simulink model "tongbukongzhi2"  (R2014b)
settings: Solver=ode45  StartTime=0.0  StopTime=10.0  RelTol=1e-3
undefined symbols (not defined in the file): sigbuilder_block
libraries: simulink x89, fuzblock x41
(part 4 of 5)

== system tongbukongzhi2/Subsystem4/Subsystem3 ==
  In4 : Inport
  In1 : Inport  Port=2
  In2 : Inport  Port=3
  In3 : Inport  Port=4
  Add : Sum  Inputs=+++
  PID Controller1 : simulink/Continuous/PID Controller  Controller=PID  TimeDomain=Continuous-time  SampleTime=-1  IntegratorMethod=Forward Euler  FilterMethod=Forward Euler  Form=Parallel  P=12.9851074749726  I=3.96505413373294  D=0.756963167778154  N=4061.73491108422  InitialConditionSource=internal  InitialConditionForIntegrator=0  InitialConditionForFilter=0  ExternalReset=none  LimitOutput=off  UpperSaturationLimit=inf  LowerSaturationLimit=-inf  LinearizeAsGain=on  AntiWindupMode=none  Kb=1  TrackingMode=off  Kt=1  PParamMin=[]  PParamMax=[]  IParamMin=[]  IParamMax=[]  DParamMin=[]  DParamMax=[]  NParamMin=[]  NParamMax=[]  KbParamMin=[]  KbParamMax=[]  KtParamMin=[]  KtParamMax=[]  POutMin=[]  POutMax=[]  IOutMin=[]  IOutMax=[]  DOutMin=[]  DOutMax=[]  NOutMin=[]  NOutMax=[]  KbOutMin=[]  KbOutMax=[]  KtOutMin=[]  KtOutMax=[]  IntegratorOutMin=[]  IntegratorOutMax=[]  FilterOutMin=[]  FilterOutMax=[]  SumOutMin=[]  SumOutMax=[]  SumI1OutMin=[]  SumI1OutMax=[]  SumI2OutMin=[]  SumI2OutMax=[]  SumI3OutMin=[]  SumI3OutMax=[]  SumDOutMin=[]  SumDOutMax=[]  SaturationOutMin=[]  SaturationOutMax=[]  IntegratorContinuousStateAttributes=''  IntegratorStateMustResolveToSignalObject=off  IntegratorRTWStateStorageClass=Auto  FilterContinuousStateAttributes=''  FilterStateMustResolveToSignalObject=off  FilterRTWStateStorageClass=Auto  DifferentiatorICPrevScaledInput=0  DifferentiatorOutMin=[]  DifferentiatorOutMax=[]  UseFilter=on
  PID Controller2 : simulink/Continuous/PID Controller  Controller=PID  TimeDomain=Continuous-time  SampleTime=-1  IntegratorMethod=Forward Euler  FilterMethod=Forward Euler  Form=Parallel  P=12.9851074749726  I=3.96505413373294  D=0.756963167778154  N=4061.73491108422  InitialConditionSource=internal  InitialConditionForIntegrator=0  InitialConditionForFilter=0  ExternalReset=none  LimitOutput=off  UpperSaturationLimit=inf  LowerSaturationLimit=-inf  LinearizeAsGain=on  AntiWindupMode=none  Kb=1  TrackingMode=off  Kt=1  PParamMin=[]  PParamMax=[]  IParamMin=[]  IParamMax=[]  DParamMin=[]  DParamMax=[]  NParamMin=[]  NParamMax=[]  KbParamMin=[]  KbParamMax=[]  KtParamMin=[]  KtParamMax=[]  POutMin=[]  POutMax=[]  IOutMin=[]  IOutMax=[]  DOutMin=[]  DOutMax=[]  NOutMin=[]  NOutMax=[]  KbOutMin=[]  KbOutMax=[]  KtOutMin=[]  KtOutMax=[]  IntegratorOutMin=[]  IntegratorOutMax=[]  FilterOutMin=[]  FilterOutMax=[]  SumOutMin=[]  SumOutMax=[]  SumI1OutMin=[]  SumI1OutMax=[]  SumI2OutMin=[]  SumI2OutMax=[]  SumI3OutMin=[]  SumI3OutMax=[]  SumDOutMin=[]  SumDOutMax=[]  SaturationOutMin=[]  SaturationOutMax=[]  IntegratorContinuousStateAttributes=''  IntegratorStateMustResolveToSignalObject=off  IntegratorRTWStateStorageClass=Auto  FilterContinuousStateAttributes=''  FilterStateMustResolveToSignalObject=off  FilterRTWStateStorageClass=Auto  DifferentiatorICPrevScaledInput=0  DifferentiatorOutMin=[]  DifferentiatorOutMax=[]  UseFilter=on
  PID Controller5 : simulink/Continuous/PID Controller  Controller=PID  TimeDomain=Continuous-time  SampleTime=-1  IntegratorMethod=Forward Euler  FilterMethod=Forward Euler  Form=Parallel  P=12.9851074749726  I=3.96505413373294  D=0.756963167778154  N=4061.73491108422  InitialConditionSource=internal  InitialConditionForIntegrator=0  InitialConditionForFilter=0  ExternalReset=none  LimitOutput=off  UpperSaturationLimit=inf  LowerSaturationLimit=-inf  LinearizeAsGain=on  AntiWindupMode=none  Kb=1  TrackingMode=off  Kt=1  PParamMin=[]  PParamMax=[]  IParamMin=[]  IParamMax=[]  DParamMin=[]  DParamMax=[]  NParamMin=[]  NParamMax=[]  KbParamMin=[]  KbParamMax=[]  KtParamMin=[]  KtParamMax=[]  POutMin=[]  POutMax=[]  IOutMin=[]  IOutMax=[]  DOutMin=[]  DOutMax=[]  NOutMin=[]  NOutMax=[]  KbOutMin=[]  KbOutMax=[]  KtOutMin=[]  KtOutMax=[]  IntegratorOutMin=[]  IntegratorOutMax=[]  FilterOutMin=[]  FilterOutMax=[]  SumOutMin=[]  SumOutMax=[]  SumI1OutMin=[]  SumI1OutMax=[]  SumI2OutMin=[]  SumI2OutMax=[]  SumI3OutMin=[]  SumI3OutMax=[]  SumDOutMin=[]  SumDOutMax=[]  SaturationOutMin=[]  SaturationOutMax=[]  IntegratorContinuousStateAttributes=''  IntegratorStateMustResolveToSignalObject=off  IntegratorRTWStateStorageClass=Auto  FilterContinuousStateAttributes=''  FilterStateMustResolveToSignalObject=off  FilterRTWStateStorageClass=Auto  DifferentiatorICPrevScaledInput=0  DifferentiatorOutMin=[]  DifferentiatorOutMax=[]  UseFilter=on
  Sum : Sum  Inputs=|+-
  Sum1 : Sum  Inputs=|+-
  Sum2 : Sum  Inputs=|+-
  Out1 : Outport
  wires:
  In4/1 -> Sum/1, Sum1/1, Sum2/1
  In1/1 -> Sum/2
  In2/1 -> Sum1/2
  In3/1 -> Sum2/2
  Sum/1 -> PID Controller1/1
  Sum1/1 -> PID Controller2/1
  Sum2/1 -> PID Controller5/1
  Add/1 -> Out1/1
  PID Controller1/1 -> Add/1
  PID Controller5/1 -> Add/3
  PID Controller2/1 -> Add/2

== system tongbukongzhi2/Subsystem4/Subsystem4 ==
  In1 : Inport
  In2 : Inport  Port=2
  In3 : Inport  Port=3
  In4 : Inport  Port=4
  Add : Sum  Inputs=+++
  PID Controller3 : simulink/Continuous/PID Controller  Controller=PID  TimeDomain=Continuous-time  SampleTime=-1  IntegratorMethod=Forward Euler  FilterMethod=Forward Euler  Form=Parallel  P=27.9924596461686  I=402.197520204602  D=0.419640505495117  N=400.016333492829  InitialConditionSource=internal  InitialConditionForIntegrator=0  InitialConditionForFilter=0  ExternalReset=none  LimitOutput=off  UpperSaturationLimit=inf  LowerSaturationLimit=-inf  LinearizeAsGain=on  AntiWindupMode=none  Kb=1  TrackingMode=off  Kt=1  PParamMin=[]  PParamMax=[]  IParamMin=[]  IParamMax=[]  DParamMin=[]  DParamMax=[]  NParamMin=[]  NParamMax=[]  KbParamMin=[]  KbParamMax=[]  KtParamMin=[]  KtParamMax=[]  POutMin=[]  POutMax=[]  IOutMin=[]  IOutMax=[]  DOutMin=[]  DOutMax=[]  NOutMin=[]  NOutMax=[]  KbOutMin=[]  KbOutMax=[]  KtOutMin=[]  KtOutMax=[]  IntegratorOutMin=[]  IntegratorOutMax=[]  FilterOutMin=[]  FilterOutMax=[]  SumOutMin=[]  SumOutMax=[]  SumI1OutMin=[]  SumI1OutMax=[]  SumI2OutMin=[]  SumI2OutMax=[]  SumI3OutMin=[]  SumI3OutMax=[]  SumDOutMin=[]  SumDOutMax=[]  SaturationOutMin=[]  SaturationOutMax=[]  IntegratorContinuousStateAttributes=''  IntegratorStateMustResolveToSignalObject=off  IntegratorRTWStateStorageClass=Auto  FilterContinuousStateAttributes=''  FilterStateMustResolveToSignalObject=off  FilterRTWStateStorageClass=Auto  DifferentiatorICPrevScaledInput=0  DifferentiatorOutMin=[]  DifferentiatorOutMax=[]  UseFilter=on
  PID Controller4 : simulink/Continuous/PID Controller  Controller=PID  TimeDomain=Continuous-time  SampleTime=-1  IntegratorMethod=Forward Euler  FilterMethod=Forward Euler  Form=Parallel  P=27.9924596461686  I=402.197520204602  D=0.419640505495117  N=400.016333492829  InitialConditionSource=internal  InitialConditionForIntegrator=0  InitialConditionForFilter=0  ExternalReset=none  LimitOutput=off  UpperSaturationLimit=inf  LowerSaturationLimit=-inf  LinearizeAsGain=on  AntiWindupMode=none  Kb=1  TrackingMode=off  Kt=1  PParamMin=[]  PParamMax=[]  IParamMin=[]  IParamMax=[]  DParamMin=[]  DParamMax=[]  NParamMin=[]  NParamMax=[]  KbParamMin=[]  KbParamMax=[]  KtParamMin=[]  KtParamMax=[]  POutMin=[]  POutMax=[]  IOutMin=[]  IOutMax=[]  DOutMin=[]  DOutMax=[]  NOutMin=[]  NOutMax=[]  KbOutMin=[]  KbOutMax=[]  KtOutMin=[]  KtOutMax=[]  IntegratorOutMin=[]  IntegratorOutMax=[]  FilterOutMin=[]  FilterOutMax=[]  SumOutMin=[]  SumOutMax=[]  SumI1OutMin=[]  SumI1OutMax=[]  SumI2OutMin=[]  SumI2OutMax=[]  SumI3OutMin=[]  SumI3OutMax=[]  SumDOutMin=[]  SumDOutMax=[]  SaturationOutMin=[]  SaturationOutMax=[]  IntegratorContinuousStateAttributes=''  IntegratorStateMustResolveToSignalObject=off  IntegratorRTWStateStorageClass=Auto  FilterContinuousStateAttributes=''  FilterStateMustResolveToSignalObject=off  FilterRTWStateStorageClass=Auto  DifferentiatorICPrevScaledInput=0  DifferentiatorOutMin=[]  DifferentiatorOutMax=[]  UseFilter=on
  PID Controller6 : simulink/Continuous/PID Controller  Controller=PID  TimeDomain=Continuous-time  SampleTime=-1  IntegratorMethod=Forward Euler  FilterMethod=Forward Euler  Form=Parallel  P=27.9924596461686  I=402.197520204602  D=0.419640505495117  N=400.016333492829  InitialConditionSource=internal  InitialConditionForIntegrator=0  InitialConditionForFilter=0  ExternalReset=none  LimitOutput=off  UpperSaturationLimit=inf  LowerSaturationLimit=-inf  LinearizeAsGain=on  AntiWindupMode=none  Kb=1  TrackingMode=off  Kt=1  PParamMin=[]  PParamMax=[]  IParamMin=[]  IParamMax=[]  DParamMin=[]  DParamMax=[]  NParamMin=[]  NParamMax=[]  KbParamMin=[]  KbParamMax=[]  KtParamMin=[]  KtParamMax=[]  POutMin=[]  POutMax=[]  IOutMin=[]  IOutMax=[]  DOutMin=[]  DOutMax=[]  NOutMin=[]  NOutMax=[]  KbOutMin=[]  KbOutMax=[]  KtOutMin=[]  KtOutMax=[]  IntegratorOutMin=[]  IntegratorOutMax=[]  FilterOutMin=[]  FilterOutMax=[]  SumOutMin=[]  SumOutMax=[]  SumI1OutMin=[]  SumI1OutMax=[]  SumI2OutMin=[]  SumI2OutMax=[]  SumI3OutMin=[]  SumI3OutMax=[]  SumDOutMin=[]  SumDOutMax=[]  SaturationOutMin=[]  SaturationOutMax=[]  IntegratorContinuousStateAttributes=''  IntegratorStateMustResolveToSignalObject=off  IntegratorRTWStateStorageClass=Auto  FilterContinuousStateAttributes=''  FilterStateMustResolveToSignalObject=off  FilterRTWStateStorageClass=Auto  DifferentiatorICPrevScaledInput=0  DifferentiatorOutMin=[]  DifferentiatorOutMax=[]  UseFilter=on
  Sum : Sum  Inputs=|+-
  Sum1 : Sum  Inputs=|+-
  Sum2 : Sum  Inputs=|+-
  Out1 : Outport
  wires:
  In1/1 -> Sum/1, Sum1/1, Sum2/1
  In2/1 -> Sum/2
  In3/1 -> Sum1/2
  In4/1 -> Sum2/2
  Sum/1 -> PID Controller3/1
  Sum1/1 -> PID Controller4/1
  Sum2/1 -> PID Controller6/1
  Add/1 -> Out1/1
  PID Controller3/1 -> Add/1
  PID Controller4/1 -> Add/2
  PID Controller6/1 -> Add/3

== system tongbukongzhi2/Subsystem4/Subsystem5 ==
  In2 : Inport
  In1 : Inport  Port=2
  In3 : Inport  Port=3
  In4 : Inport  Port=4
  Add : Sum  Inputs=+++
  PID Controller1 : simulink/Continuous/PID Controller  Controller=PID  TimeDomain=Continuous-time  SampleTime=-1  IntegratorMethod=Forward Euler  FilterMethod=Forward Euler  Form=Parallel  P=27.9924596461686  I=402.197520204602  D=0.419640505495117  N=400.016333492829  InitialConditionSource=internal  InitialConditionForIntegrator=0  InitialConditionForFilter=0  ExternalReset=none  LimitOutput=off  UpperSaturationLimit=inf  LowerSaturationLimit=-inf  LinearizeAsGain=on  AntiWindupMode=none  Kb=1  TrackingMode=off  Kt=1  PParamMin=[]  PParamMax=[]  IParamMin=[]  IParamMax=[]  DParamMin=[]  DParamMax=[]  NParamMin=[]  NParamMax=[]  KbParamMin=[]  KbParamMax=[]  KtParamMin=[]  KtParamMax=[]  POutMin=[]  POutMax=[]  IOutMin=[]  IOutMax=[]  DOutMin=[]  DOutMax=[]  NOutMin=[]  NOutMax=[]  KbOutMin=[]  KbOutMax=[]  KtOutMin=[]  KtOutMax=[]  IntegratorOutMin=[]  IntegratorOutMax=[]  FilterOutMin=[]  FilterOutMax=[]  SumOutMin=[]  SumOutMax=[]  SumI1OutMin=[]  SumI1OutMax=[]  SumI2OutMin=[]  SumI2OutMax=[]  SumI3OutMin=[]  SumI3OutMax=[]  SumDOutMin=[]  SumDOutMax=[]  SaturationOutMin=[]  SaturationOutMax=[]  IntegratorContinuousStateAttributes=''  IntegratorStateMustResolveToSignalObject=off  IntegratorRTWStateStorageClass=Auto  FilterContinuousStateAttributes=''  FilterStateMustResolveToSignalObject=off  FilterRTWStateStorageClass=Auto  DifferentiatorICPrevScaledInput=0  DifferentiatorOutMin=[]  DifferentiatorOutMax=[]  UseFilter=on
  PID Controller2 : simulink/Continuous/PID Controller  Controller=PID  TimeDomain=Continuous-time  SampleTime=-1  IntegratorMethod=Forward Euler  FilterMethod=Forward Euler  Form=Parallel  P=27.9924596461686  I=402.197520204602  D=0.419640505495117  N=400.016333492829  InitialConditionSource=internal  InitialConditionForIntegrator=0  InitialConditionForFilter=0  ExternalReset=none  LimitOutput=off  UpperSaturationLimit=inf  LowerSaturationLimit=-inf  LinearizeAsGain=on  AntiWindupMode=none  Kb=1  TrackingMode=off  Kt=1  PParamMin=[]  PParamMax=[]  IParamMin=[]  IParamMax=[]  DParamMin=[]  DParamMax=[]  NParamMin=[]  NParamMax=[]  KbParamMin=[]  KbParamMax=[]  KtParamMin=[]  KtParamMax=[]  POutMin=[]  POutMax=[]  IOutMin=[]  IOutMax=[]  DOutMin=[]  DOutMax=[]  NOutMin=[]  NOutMax=[]  KbOutMin=[]  KbOutMax=[]  KtOutMin=[]  KtOutMax=[]  IntegratorOutMin=[]  IntegratorOutMax=[]  FilterOutMin=[]  FilterOutMax=[]  SumOutMin=[]  SumOutMax=[]  SumI1OutMin=[]  SumI1OutMax=[]  SumI2OutMin=[]  SumI2OutMax=[]  SumI3OutMin=[]  SumI3OutMax=[]  SumDOutMin=[]  SumDOutMax=[]  SaturationOutMin=[]  SaturationOutMax=[]  IntegratorContinuousStateAttributes=''  IntegratorStateMustResolveToSignalObject=off  IntegratorRTWStateStorageClass=Auto  FilterContinuousStateAttributes=''  FilterStateMustResolveToSignalObject=off  FilterRTWStateStorageClass=Auto  DifferentiatorICPrevScaledInput=0  DifferentiatorOutMin=[]  DifferentiatorOutMax=[]  UseFilter=on
  PID Controller5 : simulink/Continuous/PID Controller  Controller=PID  TimeDomain=Continuous-time  SampleTime=-1  IntegratorMethod=Forward Euler  FilterMethod=Forward Euler  Form=Parallel  P=27.9924596461686  I=402.197520204602  D=0.419640505495117  N=400.016333492829  InitialConditionSource=internal  InitialConditionForIntegrator=0  InitialConditionForFilter=0  ExternalReset=none  LimitOutput=off  UpperSaturationLimit=inf  LowerSaturationLimit=-inf  LinearizeAsGain=on  AntiWindupMode=none  Kb=1  TrackingMode=off  Kt=1  PParamMin=[]  PParamMax=[]  IParamMin=[]  IParamMax=[]  DParamMin=[]  DParamMax=[]  NParamMin=[]  NParamMax=[]  KbParamMin=[]  KbParamMax=[]  KtParamMin=[]  KtParamMax=[]  POutMin=[]  POutMax=[]  IOutMin=[]  IOutMax=[]  DOutMin=[]  DOutMax=[]  NOutMin=[]  NOutMax=[]  KbOutMin=[]  KbOutMax=[]  KtOutMin=[]  KtOutMax=[]  IntegratorOutMin=[]  IntegratorOutMax=[]  FilterOutMin=[]  FilterOutMax=[]  SumOutMin=[]  SumOutMax=[]  SumI1OutMin=[]  SumI1OutMax=[]  SumI2OutMin=[]  SumI2OutMax=[]  SumI3OutMin=[]  SumI3OutMax=[]  SumDOutMin=[]  SumDOutMax=[]  SaturationOutMin=[]  SaturationOutMax=[]  IntegratorContinuousStateAttributes=''  IntegratorStateMustResolveToSignalObject=off  IntegratorRTWStateStorageClass=Auto  FilterContinuousStateAttributes=''  FilterStateMustResolveToSignalObject=off  FilterRTWStateStorageClass=Auto  DifferentiatorICPrevScaledInput=0  DifferentiatorOutMin=[]  DifferentiatorOutMax=[]  UseFilter=on
  Sum : Sum  Inputs=|+-
  Sum1 : Sum  Inputs=|+-
  Sum2 : Sum  Inputs=|+-
  Out1 : Outport
  wires:
  In2/1 -> Sum/1, Sum1/1, Sum2/1
  In1/1 -> Sum/2
  In3/1 -> Sum1/2
  In4/1 -> Sum2/2
  Sum/1 -> PID Controller1/1
  Sum1/1 -> PID Controller2/1
  Sum2/1 -> PID Controller5/1
  Add/1 -> Out1/1
  PID Controller1/1 -> Add/1
  PID Controller2/1 -> Add/2
  PID Controller5/1 -> Add/3

== system tongbukongzhi2/Subsystem4/Subsystem6 ==
  In3 : Inport
  In1 : Inport  Port=2
  In2 : Inport  Port=3
  In4 : Inport  Port=4
  Add : Sum  Inputs=+++
  PID Controller1 : simulink/Continuous/PID Controller  Controller=PID  TimeDomain=Continuous-time  SampleTime=-1  IntegratorMethod=Forward Euler  FilterMethod=Forward Euler  Form=Parallel  P=27.9924596461686  I=402.197520204602  D=0.419640505495117  N=400.016333492829  InitialConditionSource=internal  InitialConditionForIntegrator=0  InitialConditionForFilter=0  ExternalReset=none  LimitOutput=off  UpperSaturationLimit=inf  LowerSaturationLimit=-inf  LinearizeAsGain=on  AntiWindupMode=none  Kb=1  TrackingMode=off  Kt=1  PParamMin=[]  PParamMax=[]  IParamMin=[]  IParamMax=[]  DParamMin=[]  DParamMax=[]  NParamMin=[]  NParamMax=[]  KbParamMin=[]  KbParamMax=[]  KtParamMin=[]  KtParamMax=[]  POutMin=[]  POutMax=[]  IOutMin=[]  IOutMax=[]  DOutMin=[]  DOutMax=[]  NOutMin=[]  NOutMax=[]  KbOutMin=[]  KbOutMax=[]  KtOutMin=[]  KtOutMax=[]  IntegratorOutMin=[]  IntegratorOutMax=[]  FilterOutMin=[]  FilterOutMax=[]  SumOutMin=[]  SumOutMax=[]  SumI1OutMin=[]  SumI1OutMax=[]  SumI2OutMin=[]  SumI2OutMax=[]  SumI3OutMin=[]  SumI3OutMax=[]  SumDOutMin=[]  SumDOutMax=[]  SaturationOutMin=[]  SaturationOutMax=[]  IntegratorContinuousStateAttributes=''  IntegratorStateMustResolveToSignalObject=off  IntegratorRTWStateStorageClass=Auto  FilterContinuousStateAttributes=''  FilterStateMustResolveToSignalObject=off  FilterRTWStateStorageClass=Auto  DifferentiatorICPrevScaledInput=0  DifferentiatorOutMin=[]  DifferentiatorOutMax=[]  UseFilter=on
  PID Controller2 : simulink/Continuous/PID Controller  Controller=PID  TimeDomain=Continuous-time  SampleTime=-1  IntegratorMethod=Forward Euler  FilterMethod=Forward Euler  Form=Parallel  P=27.9924596461686  I=402.197520204602  D=0.419640505495117  N=400.016333492829  InitialConditionSource=internal  InitialConditionForIntegrator=0  InitialConditionForFilter=0  ExternalReset=none  LimitOutput=off  UpperSaturationLimit=inf  LowerSaturationLimit=-inf  LinearizeAsGain=on  AntiWindupMode=none  Kb=1  TrackingMode=off  Kt=1  PParamMin=[]  PParamMax=[]  IParamMin=[]  IParamMax=[]  DParamMin=[]  DParamMax=[]  NParamMin=[]  NParamMax=[]  KbParamMin=[]  KbParamMax=[]  KtParamMin=[]  KtParamMax=[]  POutMin=[]  POutMax=[]  IOutMin=[]  IOutMax=[]  DOutMin=[]  DOutMax=[]  NOutMin=[]  NOutMax=[]  KbOutMin=[]  KbOutMax=[]  KtOutMin=[]  KtOutMax=[]  IntegratorOutMin=[]  IntegratorOutMax=[]  FilterOutMin=[]  FilterOutMax=[]  SumOutMin=[]  SumOutMax=[]  SumI1OutMin=[]  SumI1OutMax=[]  SumI2OutMin=[]  SumI2OutMax=[]  SumI3OutMin=[]  SumI3OutMax=[]  SumDOutMin=[]  SumDOutMax=[]  SaturationOutMin=[]  SaturationOutMax=[]  IntegratorContinuousStateAttributes=''  IntegratorStateMustResolveToSignalObject=off  IntegratorRTWStateStorageClass=Auto  FilterContinuousStateAttributes=''  FilterStateMustResolveToSignalObject=off  FilterRTWStateStorageClass=Auto  DifferentiatorICPrevScaledInput=0  DifferentiatorOutMin=[]  DifferentiatorOutMax=[]  UseFilter=on
  PID Controller3 : simulink/Continuous/PID Controller  Controller=PID  TimeDomain=Continuous-time  SampleTime=-1  IntegratorMethod=Forward Euler  FilterMethod=Forward Euler  Form=Parallel  P=27.9924596461686  I=402.197520204602  D=0.419640505495117  N=400.016333492829  InitialConditionSource=internal  InitialConditionForIntegrator=0  InitialConditionForFilter=0  ExternalReset=none  LimitOutput=off  UpperSaturationLimit=inf  LowerSaturationLimit=-inf  LinearizeAsGain=on  AntiWindupMode=none  Kb=1  TrackingMode=off  Kt=1  PParamMin=[]  PParamMax=[]  IParamMin=[]  IParamMax=[]  DParamMin=[]  DParamMax=[]  NParamMin=[]  NParamMax=[]  KbParamMin=[]  KbParamMax=[]  KtParamMin=[]  KtParamMax=[]  POutMin=[]  POutMax=[]  IOutMin=[]  IOutMax=[]  DOutMin=[]  DOutMax=[]  NOutMin=[]  NOutMax=[]  KbOutMin=[]  KbOutMax=[]  KtOutMin=[]  KtOutMax=[]  IntegratorOutMin=[]  IntegratorOutMax=[]  FilterOutMin=[]  FilterOutMax=[]  SumOutMin=[]  SumOutMax=[]  SumI1OutMin=[]  SumI1OutMax=[]  SumI2OutMin=[]  SumI2OutMax=[]  SumI3OutMin=[]  SumI3OutMax=[]  SumDOutMin=[]  SumDOutMax=[]  SaturationOutMin=[]  SaturationOutMax=[]  IntegratorContinuousStateAttributes=''  IntegratorStateMustResolveToSignalObject=off  IntegratorRTWStateStorageClass=Auto  FilterContinuousStateAttributes=''  FilterStateMustResolveToSignalObject=off  FilterRTWStateStorageClass=Auto  DifferentiatorICPrevScaledInput=0  DifferentiatorOutMin=[]  DifferentiatorOutMax=[]  UseFilter=on
  Sum : Sum  Inputs=|+-
  Sum1 : Sum  Inputs=|+-
  Sum2 : Sum  Inputs=|+-
  Out1 : Outport
  wires:
  In3/1 -> Sum/1, Sum1/1, Sum2/1
  In1/1 -> Sum/2
  In2/1 -> Sum1/2
  In4/1 -> Sum2/2
  Sum/1 -> PID Controller1/1
  Sum1/1 -> PID Controller2/1
  Sum2/1 -> PID Controller3/1
  Add/1 -> Out1/1
  PID Controller1/1 -> Add/1
  PID Controller2/1 -> Add/2
  PID Controller3/1 -> Add/3

== system tongbukongzhi2/Subsystem4/Subsystem7 ==
  In4 : Inport
  In1 : Inport  Port=2
  In2 : Inport  Port=3
  In3 : Inport  Port=4
  Add : Sum  Inputs=+++
  PID Controller3 : simulink/Continuous/PID Controller  Controller=PID  TimeDomain=Continuous-time  SampleTime=-1  IntegratorMethod=Forward Euler  FilterMethod=Forward Euler  Form=Parallel  P=27.9924596461686  I=402.197520204602  D=0.419640505495117  N=400.016333492829  InitialConditionSource=internal  InitialConditionForIntegrator=0  InitialConditionForFilter=0  ExternalReset=none  LimitOutput=off  UpperSaturationLimit=inf  LowerSaturationLimit=-inf  LinearizeAsGain=on  AntiWindupMode=none  Kb=1  TrackingMode=off  Kt=1  PParamMin=[]  PParamMax=[]  IParamMin=[]  IParamMax=[]  DParamMin=[]  DParamMax=[]  NParamMin=[]  NParamMax=[]  KbParamMin=[]  KbParamMax=[]  KtParamMin=[]  KtParamMax=[]  POutMin=[]  POutMax=[]  IOutMin=[]  IOutMax=[]  DOutMin=[]  DOutMax=[]  NOutMin=[]  NOutMax=[]  KbOutMin=[]  KbOutMax=[]  KtOutMin=[]  KtOutMax=[]  IntegratorOutMin=[]  IntegratorOutMax=[]  FilterOutMin=[]  FilterOutMax=[]  SumOutMin=[]  SumOutMax=[]  SumI1OutMin=[]  SumI1OutMax=[]  SumI2OutMin=[]  SumI2OutMax=[]  SumI3OutMin=[]  SumI3OutMax=[]  SumDOutMin=[]  SumDOutMax=[]  SaturationOutMin=[]  SaturationOutMax=[]  IntegratorContinuousStateAttributes=''  IntegratorStateMustResolveToSignalObject=off  IntegratorRTWStateStorageClass=Auto  FilterContinuousStateAttributes=''  FilterStateMustResolveToSignalObject=off  FilterRTWStateStorageClass=Auto  DifferentiatorICPrevScaledInput=0  DifferentiatorOutMin=[]  DifferentiatorOutMax=[]  UseFilter=on
  PID Controller4 : simulink/Continuous/PID Controller  Controller=PID  TimeDomain=Continuous-time  SampleTime=-1  IntegratorMethod=Forward Euler  FilterMethod=Forward Euler  Form=Parallel  P=27.9924596461686  I=402.197520204602  D=0.419640505495117  N=400.016333492829  InitialConditionSource=internal  InitialConditionForIntegrator=0  InitialConditionForFilter=0  ExternalReset=none  LimitOutput=off  UpperSaturationLimit=inf  LowerSaturationLimit=-inf  LinearizeAsGain=on  AntiWindupMode=none  Kb=1  TrackingMode=off  Kt=1  PParamMin=[]  PParamMax=[]  IParamMin=[]  IParamMax=[]  DParamMin=[]  DParamMax=[]  NParamMin=[]  NParamMax=[]  KbParamMin=[]  KbParamMax=[]  KtParamMin=[]  KtParamMax=[]  POutMin=[]  POutMax=[]  IOutMin=[]  IOutMax=[]  DOutMin=[]  DOutMax=[]  NOutMin=[]  NOutMax=[]  KbOutMin=[]  KbOutMax=[]  KtOutMin=[]  KtOutMax=[]  IntegratorOutMin=[]  IntegratorOutMax=[]  FilterOutMin=[]  FilterOutMax=[]  SumOutMin=[]  SumOutMax=[]  SumI1OutMin=[]  SumI1OutMax=[]  SumI2OutMin=[]  SumI2OutMax=[]  SumI3OutMin=[]  SumI3OutMax=[]  SumDOutMin=[]  SumDOutMax=[]  SaturationOutMin=[]  SaturationOutMax=[]  IntegratorContinuousStateAttributes=''  IntegratorStateMustResolveToSignalObject=off  IntegratorRTWStateStorageClass=Auto  FilterContinuousStateAttributes=''  FilterStateMustResolveToSignalObject=off  FilterRTWStateStorageClass=Auto  DifferentiatorICPrevScaledInput=0  DifferentiatorOutMin=[]  DifferentiatorOutMax=[]  UseFilter=on
  PID Controller6 : simulink/Continuous/PID Controller  Controller=PID  TimeDomain=Continuous-time  SampleTime=-1  IntegratorMethod=Forward Euler  FilterMethod=Forward Euler  Form=Parallel  P=27.9924596461686  I=402.197520204602  D=0.419640505495117  N=400.016333492829  InitialConditionSource=internal  InitialConditionForIntegrator=0  InitialConditionForFilter=0  ExternalReset=none  LimitOutput=off  UpperSaturationLimit=inf  LowerSaturationLimit=-inf  LinearizeAsGain=on  AntiWindupMode=none  Kb=1  TrackingMode=off  Kt=1  PParamMin=[]  PParamMax=[]  IParamMin=[]  IParamMax=[]  DParamMin=[]  DParamMax=[]  NParamMin=[]  NParamMax=[]  KbParamMin=[]  KbParamMax=[]  KtParamMin=[]  KtParamMax=[]  POutMin=[]  POutMax=[]  IOutMin=[]  IOutMax=[]  DOutMin=[]  DOutMax=[]  NOutMin=[]  NOutMax=[]  KbOutMin=[]  KbOutMax=[]  KtOutMin=[]  KtOutMax=[]  IntegratorOutMin=[]  IntegratorOutMax=[]  FilterOutMin=[]  FilterOutMax=[]  SumOutMin=[]  SumOutMax=[]  SumI1OutMin=[]  SumI1OutMax=[]  SumI2OutMin=[]  SumI2OutMax=[]  SumI3OutMin=[]  SumI3OutMax=[]  SumDOutMin=[]  SumDOutMax=[]  SaturationOutMin=[]  SaturationOutMax=[]  IntegratorContinuousStateAttributes=''  IntegratorStateMustResolveToSignalObject=off  IntegratorRTWStateStorageClass=Auto  FilterContinuousStateAttributes=''  FilterStateMustResolveToSignalObject=off  FilterRTWStateStorageClass=Auto  DifferentiatorICPrevScaledInput=0  DifferentiatorOutMin=[]  DifferentiatorOutMax=[]  UseFilter=on
  Sum : Sum  Inputs=|+-
  Sum1 : Sum  Inputs=|+-
  Sum2 : Sum  Inputs=|+-
  Out1 : Outport
  wires:
  In4/1 -> Sum/1, Sum1/1, Sum2/1
  In1/1 -> Sum/2
  In2/1 -> Sum1/2
  In3/1 -> Sum2/2
  Sum/1 -> PID Controller3/1
  Sum1/1 -> PID Controller4/1
  Sum2/1 -> PID Controller6/1
  Add/1 -> Out1/1
  PID Controller3/1 -> Add/1
  PID Controller6/1 -> Add/3
  PID Controller4/1 -> Add/2

== system tongbukongzhi2/Subsystem4/Subsystem8 ==
  In1 : Inport
  In2 : Inport  Port=2
  In3 : Inport  Port=3
  In4 : Inport  Port=4
  Add : Sum  Inputs=+++
  PID Controller4 : simulink/Continuous/PID Controller  Controller=PID  TimeDomain=Continuous-time  SampleTime=-1  IntegratorMethod=Forward Euler  FilterMethod=Forward Euler  Form=Parallel  P=1.70949141415732  I=21.1355731705013  D=-0.019753461495741  N=20.6090721378652  InitialConditionSource=internal  InitialConditionForIntegrator=0  InitialConditionForFilter=0  ExternalReset=none  LimitOutput=off  UpperSaturationLimit=inf  LowerSaturationLimit=-inf  LinearizeAsGain=on  AntiWindupMode=none  Kb=1  TrackingMode=off  Kt=1  PParamMin=[]  PParamMax=[]  IParamMin=[]  IParamMax=[]  DParamMin=[]  DParamMax=[]  NParamMin=[]  NParamMax=[]  KbParamMin=[]  KbParamMax=[]  KtParamMin=[]  KtParamMax=[]  POutMin=[]  POutMax=[]  IOutMin=[]  IOutMax=[]  DOutMin=[]  DOutMax=[]  NOutMin=[]  NOutMax=[]  KbOutMin=[]  KbOutMax=[]  KtOutMin=[]  KtOutMax=[]  IntegratorOutMin=[]  IntegratorOutMax=[]  FilterOutMin=[]  FilterOutMax=[]  SumOutMin=[]  SumOutMax=[]  SumI1OutMin=[]  SumI1OutMax=[]  SumI2OutMin=[]  SumI2OutMax=[]  SumI3OutMin=[]  SumI3OutMax=[]  SumDOutMin=[]  SumDOutMax=[]  SaturationOutMin=[]  SaturationOutMax=[]  IntegratorContinuousStateAttributes=''  IntegratorStateMustResolveToSignalObject=off  IntegratorRTWStateStorageClass=Auto  FilterContinuousStateAttributes=''  FilterStateMustResolveToSignalObject=off  FilterRTWStateStorageClass=Auto  DifferentiatorICPrevScaledInput=0  DifferentiatorOutMin=[]  DifferentiatorOutMax=[]  UseFilter=on
  PID Controller5 : simulink/Continuous/PID Controller  Controller=PID  TimeDomain=Continuous-time  SampleTime=-1  IntegratorMethod=Forward Euler  FilterMethod=Forward Euler  Form=Parallel  P=1.70949141415732  I=21.1355731705013  D=-0.019753461495741  N=20.6090721378652  InitialConditionSource=internal  InitialConditionForIntegrator=0  InitialConditionForFilter=0  ExternalReset=none  LimitOutput=off  UpperSaturationLimit=inf  LowerSaturationLimit=-inf  LinearizeAsGain=on  AntiWindupMode=none  Kb=1  TrackingMode=off  Kt=1  PParamMin=[]  PParamMax=[]  IParamMin=[]  IParamMax=[]  DParamMin=[]  DParamMax=[]  NParamMin=[]  NParamMax=[]  KbParamMin=[]  KbParamMax=[]  KtParamMin=[]  KtParamMax=[]  POutMin=[]  POutMax=[]  IOutMin=[]  IOutMax=[]  DOutMin=[]  DOutMax=[]  NOutMin=[]  NOutMax=[]  KbOutMin=[]  KbOutMax=[]  KtOutMin=[]  KtOutMax=[]  IntegratorOutMin=[]  IntegratorOutMax=[]  FilterOutMin=[]  FilterOutMax=[]  SumOutMin=[]  SumOutMax=[]  SumI1OutMin=[]  SumI1OutMax=[]  SumI2OutMin=[]  SumI2OutMax=[]  SumI3OutMin=[]  SumI3OutMax=[]  SumDOutMin=[]  SumDOutMax=[]  SaturationOutMin=[]  SaturationOutMax=[]  IntegratorContinuousStateAttributes=''  IntegratorStateMustResolveToSignalObject=off  IntegratorRTWStateStorageClass=Auto  FilterContinuousStateAttributes=''  FilterStateMustResolveToSignalObject=off  FilterRTWStateStorageClass=Auto  DifferentiatorICPrevScaledInput=0  DifferentiatorOutMin=[]  DifferentiatorOutMax=[]  UseFilter=on
  PID Controller6 : simulink/Continuous/PID Controller  Controller=PID  TimeDomain=Continuous-time  SampleTime=-1  IntegratorMethod=Forward Euler  FilterMethod=Forward Euler  Form=Parallel  P=1.70949141415732  I=21.1355731705013  D=-0.019753461495741  N=20.6090721378652  InitialConditionSource=internal  InitialConditionForIntegrator=0  InitialConditionForFilter=0  ExternalReset=none  LimitOutput=off  UpperSaturationLimit=inf  LowerSaturationLimit=-inf  LinearizeAsGain=on  AntiWindupMode=none  Kb=1  TrackingMode=off  Kt=1  PParamMin=[]  PParamMax=[]  IParamMin=[]  IParamMax=[]  DParamMin=[]  DParamMax=[]  NParamMin=[]  NParamMax=[]  KbParamMin=[]  KbParamMax=[]  KtParamMin=[]  KtParamMax=[]  POutMin=[]  POutMax=[]  IOutMin=[]  IOutMax=[]  DOutMin=[]  DOutMax=[]  NOutMin=[]  NOutMax=[]  KbOutMin=[]  KbOutMax=[]  KtOutMin=[]  KtOutMax=[]  IntegratorOutMin=[]  IntegratorOutMax=[]  FilterOutMin=[]  FilterOutMax=[]  SumOutMin=[]  SumOutMax=[]  SumI1OutMin=[]  SumI1OutMax=[]  SumI2OutMin=[]  SumI2OutMax=[]  SumI3OutMin=[]  SumI3OutMax=[]  SumDOutMin=[]  SumDOutMax=[]  SaturationOutMin=[]  SaturationOutMax=[]  IntegratorContinuousStateAttributes=''  IntegratorStateMustResolveToSignalObject=off  IntegratorRTWStateStorageClass=Auto  FilterContinuousStateAttributes=''  FilterStateMustResolveToSignalObject=off  FilterRTWStateStorageClass=Auto  DifferentiatorICPrevScaledInput=0  DifferentiatorOutMin=[]  DifferentiatorOutMax=[]  UseFilter=on
  Sum : Sum  Inputs=|+-
  Sum1 : Sum  Inputs=|+-
  Sum2 : Sum  Inputs=|+-
  Out1 : Outport
  wires:
  In1/1 -> Sum/1, Sum1/1, Sum2/1
  In2/1 -> Sum/2
  In3/1 -> Sum1/2
  In4/1 -> Sum2/2
  Sum/1 -> PID Controller4/1
  Sum1/1 -> PID Controller5/1
  Sum2/1 -> PID Controller6/1
  Add/1 -> Out1/1
  PID Controller4/1 -> Add/1
  PID Controller5/1 -> Add/2
  PID Controller6/1 -> Add/3

== system tongbukongzhi2/Subsystem4/Subsystem9 ==
  In2 : Inport
  In1 : Inport  Port=2
  In3 : Inport  Port=3
  In4 : Inport  Port=4
  Add : Sum  Inputs=+++
  PID Controller4 : simulink/Continuous/PID Controller  Controller=PID  TimeDomain=Continuous-time  SampleTime=-1  IntegratorMethod=Forward Euler  FilterMethod=Forward Euler  Form=Parallel  P=1.70949141415732  I=21.1355731705013  D=-0.019753461495741  N=20.6090721378652  InitialConditionSource=internal  InitialConditionForIntegrator=0  InitialConditionForFilter=0  ExternalReset=none  LimitOutput=off  UpperSaturationLimit=inf  LowerSaturationLimit=-inf  LinearizeAsGain=on  AntiWindupMode=none  Kb=1  TrackingMode=off  Kt=1  PParamMin=[]  PParamMax=[]  IParamMin=[]  IParamMax=[]  DParamMin=[]  DParamMax=[]  NParamMin=[]  NParamMax=[]  KbParamMin=[]  KbParamMax=[]  KtParamMin=[]  KtParamMax=[]  POutMin=[]  POutMax=[]  IOutMin=[]  IOutMax=[]  DOutMin=[]  DOutMax=[]  NOutMin=[]  NOutMax=[]  KbOutMin=[]  KbOutMax=[]  KtOutMin=[]  KtOutMax=[]  IntegratorOutMin=[]  IntegratorOutMax=[]  FilterOutMin=[]  FilterOutMax=[]  SumOutMin=[]  SumOutMax=[]  SumI1OutMin=[]  SumI1OutMax=[]  SumI2OutMin=[]  SumI2OutMax=[]  SumI3OutMin=[]  SumI3OutMax=[]  SumDOutMin=[]  SumDOutMax=[]  SaturationOutMin=[]  SaturationOutMax=[]  IntegratorContinuousStateAttributes=''  IntegratorStateMustResolveToSignalObject=off  IntegratorRTWStateStorageClass=Auto  FilterContinuousStateAttributes=''  FilterStateMustResolveToSignalObject=off  FilterRTWStateStorageClass=Auto  DifferentiatorICPrevScaledInput=0  DifferentiatorOutMin=[]  DifferentiatorOutMax=[]  UseFilter=on
  PID Controller5 : simulink/Continuous/PID Controller  Controller=PID  TimeDomain=Continuous-time  SampleTime=-1  IntegratorMethod=Forward Euler  FilterMethod=Forward Euler  Form=Parallel  P=1.70949141415732  I=21.1355731705013  D=-0.019753461495741  N=20.6090721378652  InitialConditionSource=internal  InitialConditionForIntegrator=0  InitialConditionForFilter=0  ExternalReset=none  LimitOutput=off  UpperSaturationLimit=inf  LowerSaturationLimit=-inf  LinearizeAsGain=on  AntiWindupMode=none  Kb=1  TrackingMode=off  Kt=1  PParamMin=[]  PParamMax=[]  IParamMin=[]  IParamMax=[]  DParamMin=[]  DParamMax=[]  NParamMin=[]  NParamMax=[]  KbParamMin=[]  KbParamMax=[]  KtParamMin=[]  KtParamMax=[]  POutMin=[]  POutMax=[]  IOutMin=[]  IOutMax=[]  DOutMin=[]  DOutMax=[]  NOutMin=[]  NOutMax=[]  KbOutMin=[]  KbOutMax=[]  KtOutMin=[]  KtOutMax=[]  IntegratorOutMin=[]  IntegratorOutMax=[]  FilterOutMin=[]  FilterOutMax=[]  SumOutMin=[]  SumOutMax=[]  SumI1OutMin=[]  SumI1OutMax=[]  SumI2OutMin=[]  SumI2OutMax=[]  SumI3OutMin=[]  SumI3OutMax=[]  SumDOutMin=[]  SumDOutMax=[]  SaturationOutMin=[]  SaturationOutMax=[]  IntegratorContinuousStateAttributes=''  IntegratorStateMustResolveToSignalObject=off  IntegratorRTWStateStorageClass=Auto  FilterContinuousStateAttributes=''  FilterStateMustResolveToSignalObject=off  FilterRTWStateStorageClass=Auto  DifferentiatorICPrevScaledInput=0  DifferentiatorOutMin=[]  DifferentiatorOutMax=[]  UseFilter=on
  PID Controller6 : simulink/Continuous/PID Controller  Controller=PID  TimeDomain=Continuous-time  SampleTime=-1  IntegratorMethod=Forward Euler  FilterMethod=Forward Euler  Form=Parallel  P=1.70949141415732  I=21.1355731705013  D=-0.019753461495741  N=20.6090721378652  InitialConditionSource=internal  InitialConditionForIntegrator=0  InitialConditionForFilter=0  ExternalReset=none  LimitOutput=off  UpperSaturationLimit=inf  LowerSaturationLimit=-inf  LinearizeAsGain=on  AntiWindupMode=none  Kb=1  TrackingMode=off  Kt=1  PParamMin=[]  PParamMax=[]  IParamMin=[]  IParamMax=[]  DParamMin=[]  DParamMax=[]  NParamMin=[]  NParamMax=[]  KbParamMin=[]  KbParamMax=[]  KtParamMin=[]  KtParamMax=[]  POutMin=[]  POutMax=[]  IOutMin=[]  IOutMax=[]  DOutMin=[]  DOutMax=[]  NOutMin=[]  NOutMax=[]  KbOutMin=[]  KbOutMax=[]  KtOutMin=[]  KtOutMax=[]  IntegratorOutMin=[]  IntegratorOutMax=[]  FilterOutMin=[]  FilterOutMax=[]  SumOutMin=[]  SumOutMax=[]  SumI1OutMin=[]  SumI1OutMax=[]  SumI2OutMin=[]  SumI2OutMax=[]  SumI3OutMin=[]  SumI3OutMax=[]  SumDOutMin=[]  SumDOutMax=[]  SaturationOutMin=[]  SaturationOutMax=[]  IntegratorContinuousStateAttributes=''  IntegratorStateMustResolveToSignalObject=off  IntegratorRTWStateStorageClass=Auto  FilterContinuousStateAttributes=''  FilterStateMustResolveToSignalObject=off  FilterRTWStateStorageClass=Auto  DifferentiatorICPrevScaledInput=0  DifferentiatorOutMin=[]  DifferentiatorOutMax=[]  UseFilter=on
  Sum : Sum  Inputs=|+-
  Sum1 : Sum  Inputs=|+-
  Sum2 : Sum  Inputs=|+-
  Out1 : Outport
  wires:
  In2/1 -> Sum/1, Sum1/1, Sum2/1
  In1/1 -> Sum/2
  In3/1 -> Sum1/2
  In4/1 -> Sum2/2
  Sum/1 -> PID Controller4/1
  Sum1/1 -> PID Controller5/1
  Sum2/1 -> PID Controller6/1
  Add/1 -> Out1/1
  PID Controller4/1 -> Add/1
  PID Controller5/1 -> Add/2
  PID Controller6/1 -> Add/3

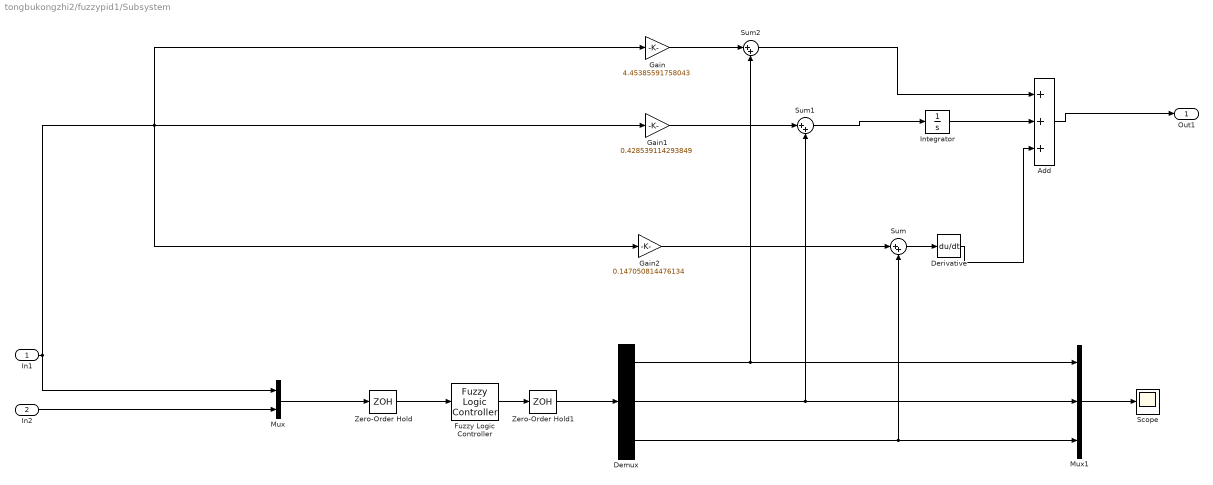
== system tongbukongzhi2/fuzzypid1/Subsystem ==
  In1 : Inport
  In2 : Inport  Port=2
  Add : Sum  Inputs=+++
  Demux : Demux  Outputs=3
  Derivative : Derivative
  Fuzzy Logic Controller : fuzblock/Fuzzy Logic  Controller  fis=fuzzy1
  Gain : Gain  Gain=4.45385591758043
  Gain1 : Gain  Gain=0.428539114293849
  Gain2 : Gain  Gain=0.147050814476134
  Integrator : Integrator
  Mux : Mux  Inputs=2
  Mux1 : Mux  Inputs=3
  Scope : Scope
      settings: SaveName=ScopeData3
  Sum : Sum  Inputs=|++
  Sum1 : Sum  Inputs=|++
  Sum2 : Sum  Inputs=|++
  Zero-Order Hold : ZeroOrderHold
  Zero-Order Hold1 : ZeroOrderHold
  Out1 : Outport
  wires:
  In1/1 -> Gain/1, Gain2/1, Gain1/1, Mux/1
  Derivative/1 -> Add/3
  Integrator/1 -> Add/2
  Add/1 -> Out1/1
  In2/1 -> Mux/2
  Gain/1 -> Sum2/1
  Sum2/1 -> Add/1
  Gain1/1 -> Sum1/1
  Sum1/1 -> Integrator/1
  Gain2/1 -> Sum/1
  Sum/1 -> Derivative/1
  Mux/1 -> Zero-Order Hold/1
  Fuzzy Logic Controller/1 -> Zero-Order Hold1/1
  Zero-Order Hold/1 -> Fuzzy Logic Controller/1
  Zero-Order Hold1/1 -> Demux/1
  Demux/1 -> Mux1/1, Sum2/2
  Demux/2 -> Mux1/2, Sum1/2
  Demux/3 -> Mux1/3, Sum/2
  Mux1/1 -> Scope/1

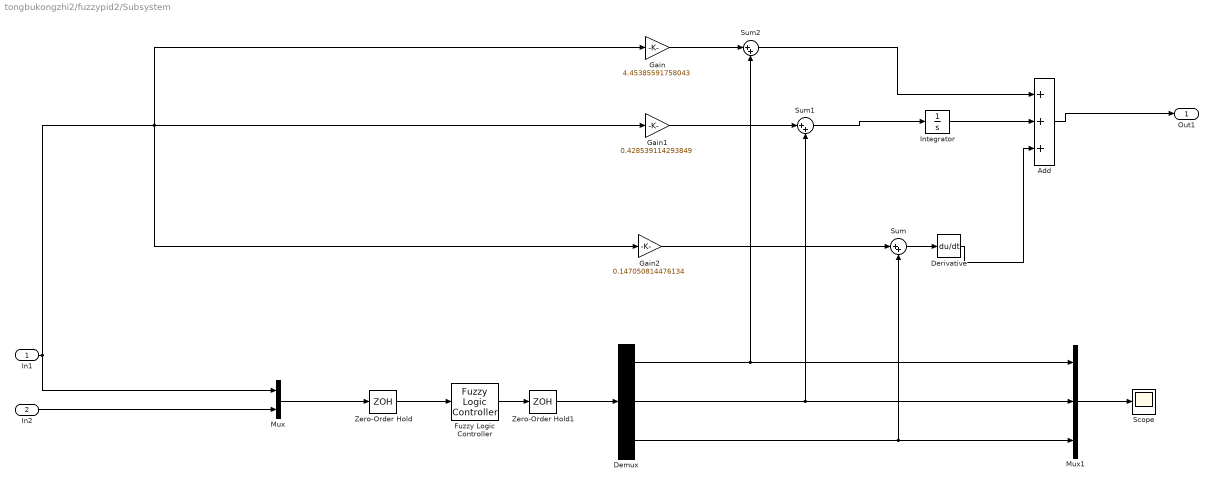
== system tongbukongzhi2/fuzzypid2/Subsystem ==
  In1 : Inport
  In2 : Inport  Port=2
  Add : Sum  Inputs=+++
  Demux : Demux  Outputs=3
  Derivative : Derivative
  Fuzzy Logic Controller : fuzblock/Fuzzy Logic  Controller  fis=fuzzy1
  Gain : Gain  Gain=4.45385591758043
  Gain1 : Gain  Gain=0.428539114293849
  Gain2 : Gain  Gain=0.147050814476134
  Integrator : Integrator
  Mux : Mux  Inputs=2
  Mux1 : Mux  Inputs=3
  Scope : Scope
      settings: SaveName=ScopeData2
  Sum : Sum  Inputs=|++
  Sum1 : Sum  Inputs=|++
  Sum2 : Sum  Inputs=|++
  Zero-Order Hold : ZeroOrderHold
  Zero-Order Hold1 : ZeroOrderHold
  Out1 : Outport
  wires:
  In1/1 -> Gain/1, Gain2/1, Gain1/1, Mux/1
  Derivative/1 -> Add/3
  Integrator/1 -> Add/2
  Add/1 -> Out1/1
  In2/1 -> Mux/2
  Gain/1 -> Sum2/1
  Sum2/1 -> Add/1
  Gain1/1 -> Sum1/1
  Sum1/1 -> Integrator/1
  Gain2/1 -> Sum/1
  Sum/1 -> Derivative/1
  Mux/1 -> Zero-Order Hold/1
  Fuzzy Logic Controller/1 -> Zero-Order Hold1/1
  Zero-Order Hold/1 -> Fuzzy Logic Controller/1
  Zero-Order Hold1/1 -> Demux/1
  Demux/1 -> Mux1/1, Sum2/2
  Demux/2 -> Mux1/2, Sum1/2
  Demux/3 -> Mux1/3, Sum/2
  Mux1/1 -> Scope/1

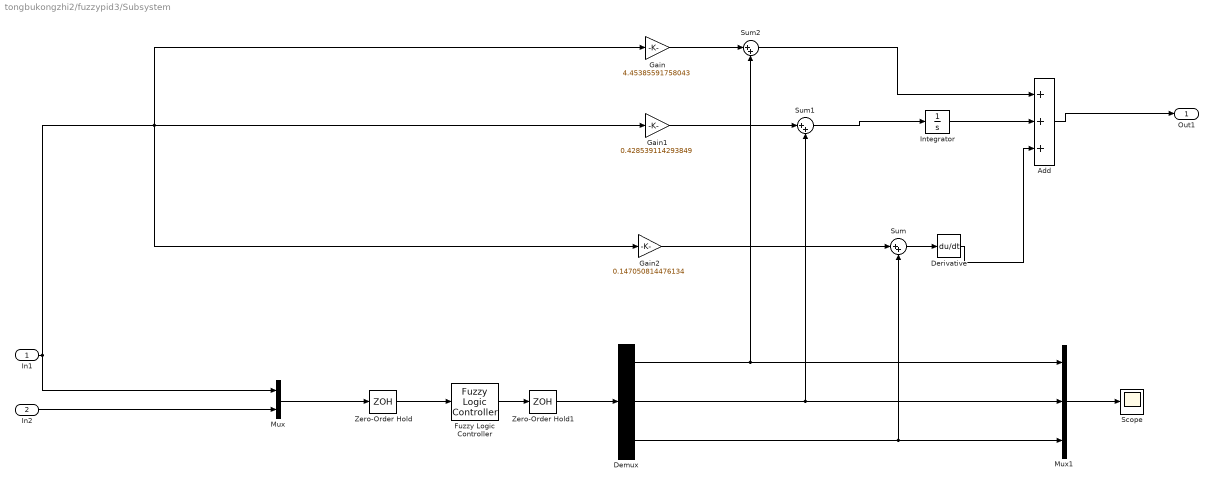
== system tongbukongzhi2/fuzzypid3/Subsystem ==
  In1 : Inport
  In2 : Inport  Port=2
  Add : Sum  Inputs=+++
  Demux : Demux  Outputs=3
  Derivative : Derivative
  Fuzzy Logic Controller : fuzblock/Fuzzy Logic  Controller  fis=fuzzy1
  Gain : Gain  Gain=4.45385591758043
  Gain1 : Gain  Gain=0.428539114293849
  Gain2 : Gain  Gain=0.147050814476134
  Integrator : Integrator
  Mux : Mux  Inputs=2
  Mux1 : Mux  Inputs=3
  Scope : Scope
  Sum : Sum  Inputs=|++
  Sum1 : Sum  Inputs=|++
  Sum2 : Sum  Inputs=|++
  Zero-Order Hold : ZeroOrderHold
  Zero-Order Hold1 : ZeroOrderHold
  Out1 : Outport
  wires:
  In1/1 -> Gain/1, Gain2/1, Gain1/1, Mux/1
  Derivative/1 -> Add/3
  Integrator/1 -> Add/2
  Add/1 -> Out1/1
  In2/1 -> Mux/2
  Gain/1 -> Sum2/1
  Sum2/1 -> Add/1
  Gain1/1 -> Sum1/1
  Sum1/1 -> Integrator/1
  Gain2/1 -> Sum/1
  Sum/1 -> Derivative/1
  Demux/1 -> Mux1/1, Sum2/2
  Demux/2 -> Sum1/2, Mux1/2
  Demux/3 -> Sum/2, Mux1/3
  Mux/1 -> Zero-Order Hold/1
  Fuzzy Logic Controller/1 -> Zero-Order Hold1/1
  Zero-Order Hold/1 -> Fuzzy Logic Controller/1
  Zero-Order Hold1/1 -> Demux/1
  Mux1/1 -> Scope/1

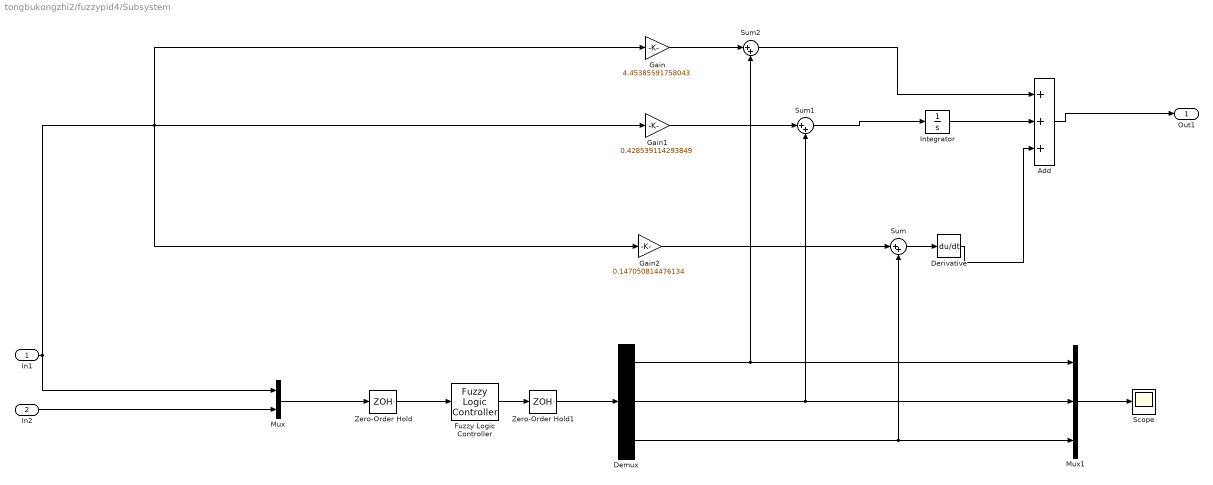
== system tongbukongzhi2/fuzzypid4/Subsystem ==
  In1 : Inport
  In2 : Inport  Port=2
  Add : Sum  Inputs=+++
  Demux : Demux  Outputs=3
  Derivative : Derivative
  Fuzzy Logic Controller : fuzblock/Fuzzy Logic  Controller  fis=fuzzy1
  Gain : Gain  Gain=4.45385591758043
  Gain1 : Gain  Gain=0.428539114293849
  Gain2 : Gain  Gain=0.147050814476134
  Integrator : Integrator
  Mux : Mux  Inputs=2
  Mux1 : Mux  Inputs=3
  Scope : Scope
  Sum : Sum  Inputs=|++
  Sum1 : Sum  Inputs=|++
  Sum2 : Sum  Inputs=|++
  Zero-Order Hold : ZeroOrderHold
  Zero-Order Hold1 : ZeroOrderHold
  Out1 : Outport
  wires:
  In1/1 -> Gain/1, Gain2/1, Gain1/1, Mux/1
  Derivative/1 -> Add/3
  Integrator/1 -> Add/2
  Add/1 -> Out1/1
  In2/1 -> Mux/2
  Gain/1 -> Sum2/1
  Sum2/1 -> Add/1
  Gain1/1 -> Sum1/1
  Sum1/1 -> Integrator/1
  Gain2/1 -> Sum/1
  Sum/1 -> Derivative/1
  Mux/1 -> Zero-Order Hold/1
  Fuzzy Logic Controller/1 -> Zero-Order Hold1/1
  Zero-Order Hold/1 -> Fuzzy Logic Controller/1
  Zero-Order Hold1/1 -> Demux/1
  Demux/1 -> Mux1/1, Sum2/2
  Demux/2 -> Mux1/2, Sum1/2
  Demux/3 -> Mux1/3, Sum/2
  Mux1/1 -> Scope/1

== system tongbukongzhi2/Subsystem1/Subsystem/fuzzypid1 ==
  In1 : Inport
  Derivative : Derivative
  Subsystem : Subsystem
  Out1 : Outport
  wires:
  Subsystem/1(Out1) -> Out1/1
  Derivative/1 -> Subsystem/2(In2)
  In1/1 -> Derivative/1, Subsystem/1(In1)

== system tongbukongzhi2/Subsystem1/Subsystem/fuzzypid2 ==
  In1 : Inport
  Derivative : Derivative
  Subsystem : Subsystem
  Out1 : Outport
  wires:
  Subsystem/1(Out1) -> Out1/1
  Derivative/1 -> Subsystem/2(In2)
  In1/1 -> Derivative/1, Subsystem/1(In1)

== system tongbukongzhi2/Subsystem1/Subsystem/fuzzypid4 ==
  In1 : Inport
  Derivative : Derivative
  Subsystem : Subsystem
  Out1 : Outport
  wires:
  Subsystem/1(Out1) -> Out1/1
  Derivative/1 -> Subsystem/2(In2)
  In1/1 -> Derivative/1, Subsystem/1(In1)

== system tongbukongzhi2/Subsystem1/Subsystem1/fuzzypid4 ==
  In1 : Inport
  Derivative : Derivative
  Subsystem : Subsystem
  Out1 : Outport
  wires:
  Subsystem/1(Out1) -> Out1/1
  Derivative/1 -> Subsystem/2(In2)
  In1/1 -> Derivative/1, Subsystem/1(In1)

== system tongbukongzhi2/Subsystem1/Subsystem1/fuzzypid5 ==
  In1 : Inport
  Derivative : Derivative
  Subsystem : Subsystem
  Out1 : Outport
  wires:
  Subsystem/1(Out1) -> Out1/1
  Derivative/1 -> Subsystem/2(In2)
  In1/1 -> Derivative/1, Subsystem/1(In1)

== system tongbukongzhi2/Subsystem1/Subsystem1/fuzzypid6 ==
  In1 : Inport
  Derivative : Derivative
  Subsystem : Subsystem
  Out1 : Outport
  wires:
  Subsystem/1(Out1) -> Out1/1
  Derivative/1 -> Subsystem/2(In2)
  In1/1 -> Derivative/1, Subsystem/1(In1)

== system tongbukongzhi2/Subsystem1/Subsystem12/fuzzypid1 ==
  In1 : Inport
  Derivative : Derivative
  Subsystem : Subsystem
  Out1 : Outport
  wires:
  Subsystem/1(Out1) -> Out1/1
  Derivative/1 -> Subsystem/2(In2)
  In1/1 -> Derivative/1, Subsystem/1(In1)

== system tongbukongzhi2/Subsystem1/Subsystem12/fuzzypid2 ==
  In1 : Inport
  Derivative : Derivative
  Subsystem : Subsystem
  Out1 : Outport
  wires:
  Subsystem/1(Out1) -> Out1/1
  Derivative/1 -> Subsystem/2(In2)
  In1/1 -> Derivative/1, Subsystem/1(In1)

== system tongbukongzhi2/Subsystem1/Subsystem12/fuzzypid3 ==
  In1 : Inport
  Derivative : Derivative
  Subsystem : Subsystem
  Out1 : Outport
  wires:
  Subsystem/1(Out1) -> Out1/1
  Derivative/1 -> Subsystem/2(In2)
  In1/1 -> Derivative/1, Subsystem/1(In1)

== system tongbukongzhi2/Subsystem1/Subsystem13/fuzzypid1 ==
  In1 : Inport
  Derivative : Derivative
  Subsystem : Subsystem
  Out1 : Outport
  wires:
  Subsystem/1(Out1) -> Out1/1
  Derivative/1 -> Subsystem/2(In2)
  In1/1 -> Derivative/1, Subsystem/1(In1)

== system tongbukongzhi2/Subsystem1/Subsystem13/fuzzypid2 ==
  In1 : Inport
  Derivative : Derivative
  Subsystem : Subsystem
  Out1 : Outport
  wires:
  Subsystem/1(Out1) -> Out1/1
  Derivative/1 -> Subsystem/2(In2)
  In1/1 -> Derivative/1, Subsystem/1(In1)

== system tongbukongzhi2/Subsystem1/Subsystem13/fuzzypid3 ==
  In1 : Inport
  Derivative : Derivative
  Subsystem : Subsystem
  Out1 : Outport
  wires:
  Subsystem/1(Out1) -> Out1/1
  Derivative/1 -> Subsystem/2(In2)
  In1/1 -> Derivative/1, Subsystem/1(In1)

== system tongbukongzhi2/Subsystem1/Subsystem14/fuzzypid1 ==
  In1 : Inport
  Derivative : Derivative
  Subsystem : Subsystem
  Out1 : Outport
  wires:
  Subsystem/1(Out1) -> Out1/1
  Derivative/1 -> Subsystem/2(In2)
  In1/1 -> Derivative/1, Subsystem/1(In1)

== system tongbukongzhi2/Subsystem1/Subsystem14/fuzzypid2 ==
  In1 : Inport
  Derivative : Derivative
  Subsystem : Subsystem
  Out1 : Outport
  wires:
  Subsystem/1(Out1) -> Out1/1
  Derivative/1 -> Subsystem/2(In2)
  In1/1 -> Derivative/1, Subsystem/1(In1)

== system tongbukongzhi2/Subsystem1/Subsystem14/fuzzypid3 ==
  In1 : Inport
  Derivative : Derivative
  Subsystem : Subsystem
  Out1 : Outport
  wires:
  Subsystem/1(Out1) -> Out1/1
  Derivative/1 -> Subsystem/2(In2)
  In1/1 -> Derivative/1, Subsystem/1(In1)

== system tongbukongzhi2/Subsystem1/Subsystem15/fuzzypid1 ==
  In1 : Inport
  Derivative : Derivative
  Subsystem : Subsystem
  Out1 : Outport
  wires:
  Subsystem/1(Out1) -> Out1/1
  Derivative/1 -> Subsystem/2(In2)
  In1/1 -> Derivative/1, Subsystem/1(In1)

== system tongbukongzhi2/Subsystem1/Subsystem15/fuzzypid2 ==
  In1 : Inport
  Derivative : Derivative
  Subsystem : Subsystem
  Out1 : Outport
  wires:
  Subsystem/1(Out1) -> Out1/1
  Derivative/1 -> Subsystem/2(In2)
  In1/1 -> Derivative/1, Subsystem/1(In1)

== system tongbukongzhi2/Subsystem1/Subsystem15/fuzzypid3 ==
  In1 : Inport
  Derivative : Derivative
  Subsystem : Subsystem
  Out1 : Outport
  wires:
  Subsystem/1(Out1) -> Out1/1
  Derivative/1 -> Subsystem/2(In2)
  In1/1 -> Derivative/1, Subsystem/1(In1)

== system tongbukongzhi2/Subsystem1/Subsystem16/fuzzypid1 ==
  In1 : Inport
  Derivative : Derivative
  Subsystem : Subsystem
  Out1 : Outport
  wires:
  Subsystem/1(Out1) -> Out1/1
  Derivative/1 -> Subsystem/2(In2)
  In1/1 -> Derivative/1, Subsystem/1(In1)

== system tongbukongzhi2/Subsystem1/Subsystem16/fuzzypid2 ==
  In1 : Inport
  Derivative : Derivative
  Subsystem : Subsystem
  Out1 : Outport
  wires:
  Subsystem/1(Out1) -> Out1/1
  Derivative/1 -> Subsystem/2(In2)
  In1/1 -> Derivative/1, Subsystem/1(In1)

== system tongbukongzhi2/Subsystem1/Subsystem16/fuzzypid4 ==
  In1 : Inport
  Derivative : Derivative
  Subsystem : Subsystem
  Out1 : Outport
  wires:
  Subsystem/1(Out1) -> Out1/1
  Derivative/1 -> Subsystem/2(In2)
  In1/1 -> Derivative/1, Subsystem/1(In1)

== system tongbukongzhi2/Subsystem1/Subsystem17/fuzzypid4 ==
  In1 : Inport
  Derivative : Derivative
  Subsystem : Subsystem
  Out1 : Outport
  wires:
  Subsystem/1(Out1) -> Out1/1
  Derivative/1 -> Subsystem/2(In2)
  In1/1 -> Derivative/1, Subsystem/1(In1)

== system tongbukongzhi2/Subsystem1/Subsystem17/fuzzypid5 ==
  In1 : Inport
  Derivative : Derivative
  Subsystem : Subsystem
  Out1 : Outport
  wires:
  Subsystem/1(Out1) -> Out1/1
  Derivative/1 -> Subsystem/2(In2)
  In1/1 -> Derivative/1, Subsystem/1(In1)

== system tongbukongzhi2/Subsystem1/Subsystem17/fuzzypid6 ==
  In1 : Inport
  Derivative : Derivative
  Subsystem : Subsystem
  Out1 : Outport
  wires:
  Subsystem/1(Out1) -> Out1/1
  Derivative/1 -> Subsystem/2(In2)
  In1/1 -> Derivative/1, Subsystem/1(In1)

== system tongbukongzhi2/Subsystem1/Subsystem18/fuzzypid4 ==
  In1 : Inport
  Derivative : Derivative
  Subsystem : Subsystem
  Out1 : Outport
  wires:
  Subsystem/1(Out1) -> Out1/1
  Derivative/1 -> Subsystem/2(In2)
  In1/1 -> Derivative/1, Subsystem/1(In1)

== system tongbukongzhi2/Subsystem1/Subsystem18/fuzzypid5 ==
  In1 : Inport
  Derivative : Derivative
  Subsystem : Subsystem
  Out1 : Outport
  wires:
  Subsystem/1(Out1) -> Out1/1
  Derivative/1 -> Subsystem/2(In2)
  In1/1 -> Derivative/1, Subsystem/1(In1)

== system tongbukongzhi2/Subsystem1/Subsystem18/fuzzypid6 ==
  In1 : Inport
  Derivative : Derivative
  Subsystem : Subsystem
  Out1 : Outport
  wires:
  Subsystem/1(Out1) -> Out1/1
  Derivative/1 -> Subsystem/2(In2)
  In1/1 -> Derivative/1, Subsystem/1(In1)

== system tongbukongzhi2/Subsystem1/Subsystem19/fuzzypid4 ==
  In1 : Inport
  Derivative : Derivative
  Subsystem : Subsystem
  Out1 : Outport
  wires:
  Subsystem/1(Out1) -> Out1/1
  Derivative/1 -> Subsystem/2(In2)
  In1/1 -> Derivative/1, Subsystem/1(In1)

== system tongbukongzhi2/Subsystem1/Subsystem19/fuzzypid5 ==
  In1 : Inport
  Derivative : Derivative
  Subsystem : Subsystem
  Out1 : Outport
  wires:
  Subsystem/1(Out1) -> Out1/1
  Derivative/1 -> Subsystem/2(In2)
  In1/1 -> Derivative/1, Subsystem/1(In1)

== system tongbukongzhi2/Subsystem1/Subsystem19/fuzzypid6 ==
  In1 : Inport
  Derivative : Derivative
  Subsystem : Subsystem
  Out1 : Outport
  wires:
  Subsystem/1(Out1) -> Out1/1
  Derivative/1 -> Subsystem/2(In2)
  In1/1 -> Derivative/1, Subsystem/1(In1)

== system tongbukongzhi2/Subsystem1/Subsystem2/fuzzypid4 ==
  In1 : Inport
  Derivative : Derivative
  Subsystem : Subsystem
  Out1 : Outport
  wires:
  Subsystem/1(Out1) -> Out1/1
  Derivative/1 -> Subsystem/2(In2)
  In1/1 -> Derivative/1, Subsystem/1(In1)

== system tongbukongzhi2/Subsystem1/Subsystem2/fuzzypid5 ==
  In1 : Inport
  Derivative : Derivative
  Subsystem : Subsystem
  Out1 : Outport
  wires:
  Subsystem/1(Out1) -> Out1/1
  Derivative/1 -> Subsystem/2(In2)
  In1/1 -> Derivative/1, Subsystem/1(In1)

== system tongbukongzhi2/Subsystem1/Subsystem2/fuzzypid6 ==
  In1 : Inport
  Derivative : Derivative
  Subsystem : Subsystem
  Out1 : Outport
  wires:
  Subsystem/1(Out1) -> Out1/1
  Derivative/1 -> Subsystem/2(In2)
  In1/1 -> Derivative/1, Subsystem/1(In1)

== system tongbukongzhi2/Subsystem1/Subsystem3/fuzzypid4 ==
  In1 : Inport
  Derivative : Derivative
  Subsystem : Subsystem
  Out1 : Outport
  wires:
  Subsystem/1(Out1) -> Out1/1
  Derivative/1 -> Subsystem/2(In2)
  In1/1 -> Derivative/1, Subsystem/1(In1)

== system tongbukongzhi2/Subsystem1/Subsystem3/fuzzypid5 ==
  In1 : Inport
  Derivative : Derivative
  Subsystem : Subsystem
  Out1 : Outport
  wires:
  Subsystem/1(Out1) -> Out1/1
  Derivative/1 -> Subsystem/2(In2)
  In1/1 -> Derivative/1, Subsystem/1(In1)

== system tongbukongzhi2/Subsystem1/Subsystem3/fuzzypid6 ==
  In1 : Inport
  Derivative : Derivative
  Subsystem : Subsystem
  Out1 : Outport
  wires:
  Subsystem/1(Out1) -> Out1/1
  Derivative/1 -> Subsystem/2(In2)
  In1/1 -> Derivative/1, Subsystem/1(In1)

== system tongbukongzhi2/Subsystem1/Subsystem8/fuzzypid2 ==
  In1 : Inport
  Derivative : Derivative
  Subsystem : Subsystem
  Out1 : Outport
  wires:
  Subsystem/1(Out1) -> Out1/1
  Derivative/1 -> Subsystem/2(In2)
  In1/1 -> Derivative/1, Subsystem/1(In1)

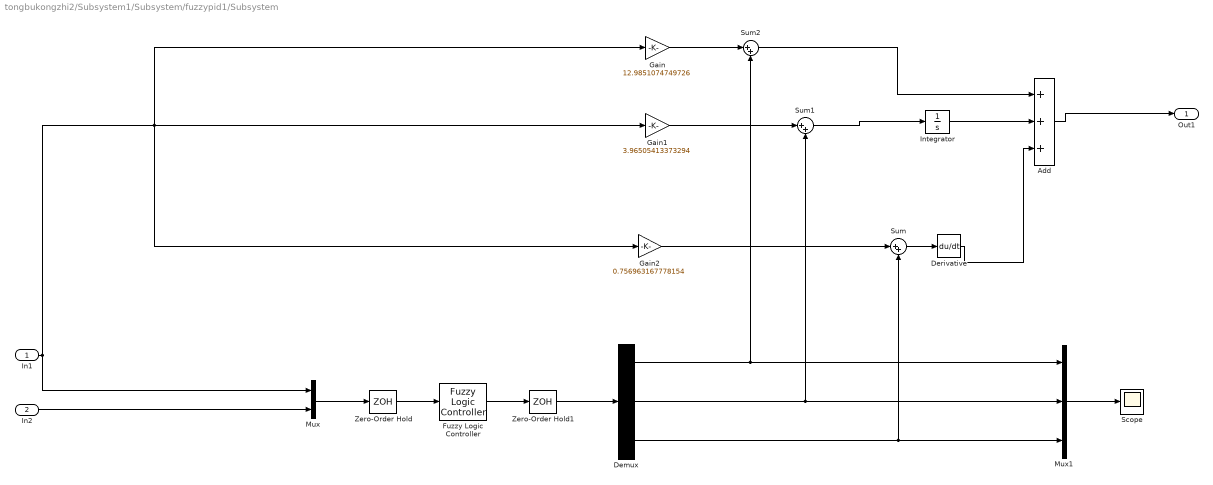
== system tongbukongzhi2/Subsystem1/Subsystem/fuzzypid1/Subsystem ==
  In1 : Inport
  In2 : Inport  Port=2
  Add : Sum  Inputs=+++
  Demux : Demux  Outputs=3
  Derivative : Derivative
  Fuzzy Logic Controller : fuzblock/Fuzzy Logic  Controller  fis=fuzzy1
  Gain : Gain  Gain=12.9851074749726
  Gain1 : Gain  Gain=3.96505413373294
  Gain2 : Gain  Gain=0.756963167778154
  Integrator : Integrator
  Mux : Mux  Inputs=2
  Mux1 : Mux  Inputs=3
  Scope : Scope
      settings: YMin=-0.2  YMax=0.05
  Sum : Sum  Inputs=|++
  Sum1 : Sum  Inputs=|++
  Sum2 : Sum  Inputs=|++
  Zero-Order Hold : ZeroOrderHold  SampleTime=0.1
  Zero-Order Hold1 : ZeroOrderHold  SampleTime=0.1
  Out1 : Outport
  wires:
  In1/1 -> Gain/1, Gain2/1, Gain1/1, Mux/1
  Derivative/1 -> Add/3
  Integrator/1 -> Add/2
  Add/1 -> Out1/1
  In2/1 -> Mux/2
  Gain/1 -> Sum2/1
  Sum2/1 -> Add/1
  Gain1/1 -> Sum1/1
  Sum1/1 -> Integrator/1
  Gain2/1 -> Sum/1
  Sum/1 -> Derivative/1
  Mux/1 -> Zero-Order Hold/1
  Fuzzy Logic Controller/1 -> Zero-Order Hold1/1
  Zero-Order Hold/1 -> Fuzzy Logic Controller/1
  Zero-Order Hold1/1 -> Demux/1
  Mux1/1 -> Scope/1
  Demux/3 -> Sum/2, Mux1/3
  Demux/2 -> Sum1/2, Mux1/2
  Demux/1 -> Mux1/1, Sum2/2
